simulink model "fastSlowModel"  (R2015a)
settings: Solver=ode45  StartTime=0.0  StopTime=3000  RelTol=1e-3
values from neighbouring files (symbols this model uses):
  alpha_const = 0.0    (= 0)    [averagedRelayOutput.m]    (also in bursting_linearised.m = 0.1; fastSlow.m = 0.1; manParamsNullclines.m; manipulateParameters.m = getappdata(hObject.Parent,'alpha_const'))
  beta = 0.37    [averagedRelayOutput.m]    (also in bursting_linearised.m = 0.27; compareApproximations.m = 1.5; fastSlow.m = 0.27; fast_nullcline_winged_cusp.m = 0.5)
  gamma = 0    [averagedRelayOutput.m]    (also in bursting_linearised.m = 1; compareApproximations.m = 1; fastSlow.m = 1; fast_nullcline_winged_cusp.m = 1)
  kb = -0.5    [averagedRelayOutput.m]    (also in fastSlow.m; findPeriodForAsymmOscill.m = 0.5; originalModel2.m; product.m)
  ts = 1    [averagedRelayOutput.m]    (also in bursting_linearised.m; compareApproximations.m; fastSlow.m; fast_nullcline_winged_cusp.m)
  tus = 800    [averagedRelayOutput.m]    (also in bursting_linearised.m; fastSlow.m; manParamsNullclines.m; manipulateParameters.m = getappdata(hObject.Parent,'tus'))
  ultra_slow_plant_X0 = 0.45    [averagedRelayOutput.m]    (also in bursting_linearised.m = 0; fastSlow.m = 0; hRose.m = 2000; manParamsNullclines.m)
settings Model: Creator=ra428  LastModifiedBy=ra428

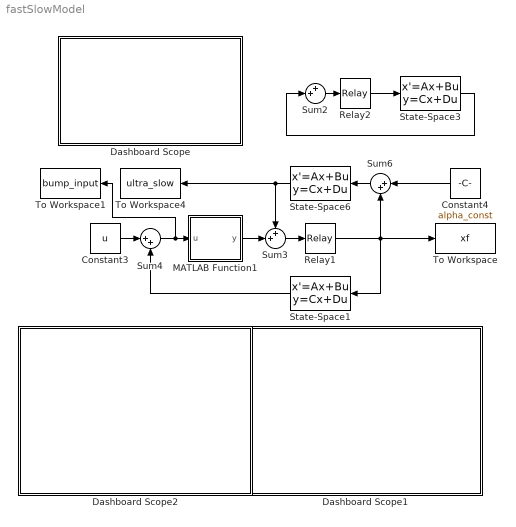
== system fastSlowModel ==
  Constant3 : Constant  Value=u
  Constant4 : Constant  Value=alpha_const
  Dashboard Scope : Subsystem  DialogController=hmiCreateDDGDialog  IsWebBlock=on  mask(MathWorksWebBlock){webBlockId=86d8a679-5039-43ce-9683-fe3f2f848e5b, webBlockType=sdiscope, ShowInitialText=on, HMISrcModelName=fastSlowModel}
      mask prompts: webBlockId "WebBlock Id"; webBlockType "WebBlock Type"; HMISrcModelName "Source Model"
      mask Help: helpview([docroot '/mapfiles/simulink.map'], 'hmi_scope')
      mask Display:
      | if strcmp(get_param(bdroot(gcb),'BlockDiagramType'), 'library')
      |     image([(matlabroot) '/toolbox/simulink/hmi/icons/DashboardScope.png']);
      | end
  Dashboard Scope1 : Subsystem  DialogController=hmiCreateDDGDialog  IsWebBlock=on  mask(MathWorksWebBlock){webBlockId=de4fc884-cf29-4a10-8f9d-8ea8cac4978b, webBlockType=sdiscope, ShowInitialText=on, HMISrcModelName=fastSlowModel}
      mask prompts: webBlockId "WebBlock Id"; webBlockType "WebBlock Type"; HMISrcModelName "Source Model"
      mask Help: helpview([docroot '/mapfiles/simulink.map'], 'hmi_scope')
      mask Display:
      | if strcmp(get_param(bdroot(gcb),'BlockDiagramType'), 'library')
      |     image([(matlabroot) '/toolbox/simulink/hmi/icons/DashboardScope.png']);
      | end
  Dashboard Scope2 : Subsystem  DialogController=hmiCreateDDGDialog  IsWebBlock=on  mask(MathWorksWebBlock){webBlockId=23221fb1-a0a9-412c-ab90-5e3ffe948c2d, webBlockType=sdiscope, ShowInitialText=on, HMISrcModelName=fastSlowModel}
      mask prompts: webBlockId "WebBlock Id"; webBlockType "WebBlock Type"; HMISrcModelName "Source Model"
      mask Help: helpview([docroot '/mapfiles/simulink.map'], 'hmi_scope')
      mask Display:
      | if strcmp(get_param(bdroot(gcb),'BlockDiagramType'), 'library')
      |     image([(matlabroot) '/toolbox/simulink/hmi/icons/DashboardScope.png']);
      | end
  MATLAB Function1 : MATLAB Function  TreatAsAtomicUnit=on
  Relay1 : Relay  OnSwitchValue=beta  OffSwitchValue=-beta  OffOutputValue=-1
  Relay2 : Relay  OnSwitchValue=beta-kb*u  OffSwitchValue=-beta-kb*u  OffOutputValue=-1
  State-Space1 : StateSpace  A=-1/ts  B=1/ts  D=0.5*1*gamma  X0=0
  State-Space3 : StateSpace  A=-1/ts  B=kb/ts  D=0.5*kb*gamma  X0=0
  State-Space6 : StateSpace  A=-1/tus  B=-1/tus  D=0  X0=ultra_slow_plant_X0
  Sum2 : Sum  Inputs=++|
  Sum3 : Sum  Inputs=++|
  Sum4 : Sum  Inputs=|++
  Sum6 : Sum  Inputs=|++
  To Workspace : ToWorkspace  VariableName=xf  SaveFormat=Timeseries  SampleTime=-1
  To Workspace1 : ToWorkspace  VariableName=bump_input  SaveFormat=Timeseries  SampleTime=-1
  To Workspace4 : ToWorkspace  VariableName=ultra_slow  SaveFormat=Timeseries  SampleTime=-1
  wires:
  Relay2/1 -> State-Space3/1
  State-Space3/1 -> Sum2/2
  Sum2/1 -> Relay2/1
  Sum3/1 -> Relay1/1
  Constant3/1 -> Sum4/1
  Relay1/1 -> Sum6/2, To Workspace/1, State-Space1/1
  State-Space1/1 -> Sum4/2
  Constant4/1 -> Sum6/1
  Sum6/1 -> State-Space6/1
  State-Space6/1 -> Sum3/1, To Workspace4/1
  MATLAB Function1/1(y) -> Sum3/2
  Sum4/1 -> To Workspace1/1, MATLAB Function1/1(u)

== system fastSlowModel/Dashboard Scope ==

== system fastSlowModel/Dashboard Scope1 ==

== system fastSlowModel/Dashboard Scope2 ==

== matlab function fastSlowModel/MATLAB Function1 ==
  data: u input; y output
function y = fcn(u)
%#codegen
if (u < -2)
    y = -1;
elseif (u > 2)
    y = -1;
elseif and( u>=-2,u < 0)
    y = 0.5*u;
else
    y = -0.5*u;
end
